simulink model "integral_backstepping"  (R2025a)
settings: Solver=VariableStepAuto  StartTime=0.0  StopTime=t_total(end)  RelTol=1e-3
StopFcn:
  | autoplot;
values from neighbouring files (symbols this model uses):
  Ib = diag([params.Ix, params.Iy, params.Iz])    [setup_mission.m]
  lin_vel_0 = [0; 0; 0]    [setup_mission.m]
  mass = params.m    [setup_mission.m]
  pos_0 = p_ref(:,1) + offset_init    [setup_mission.m]
  w_bb_0 = [0; 0; 0]    [setup_mission.m]
libraries: robotcorelib x2, uavutilslib x1
settings Model: Creator=marco  LastModifiedBy=marco

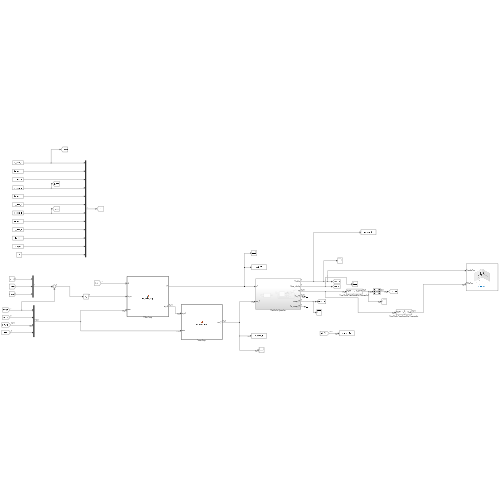
[thumbnail: Simulink's stored preview of the top-level diagram]
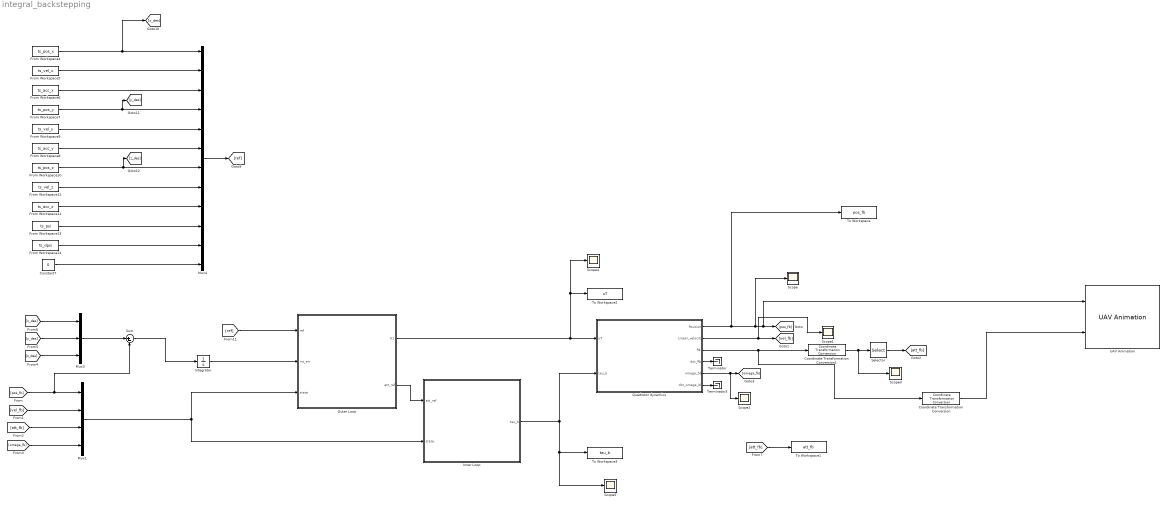
== system integral_backstepping ==
  Constant7 : Constant  Value=0
  Coordinate Transformation Conversion : robotcorelib/Coordinate Transformation Conversion  InputRepresentation=Rotation Matrix  InputEulerSequence=ZYX  ShowTrVecInputPort=on  OutputRepresentation=Quaternion  OutputEulerSequence=ZYX  ShowTrVecOutputPort=on  SimulateUsing=Interpreted execution
  Coordinate Transformation Conversion1 : robotcorelib/Coordinate Transformation Conversion  InputRepresentation=Rotation Matrix  InputEulerSequence=ZYX  ShowTrVecInputPort=on  OutputRepresentation=Euler Angles  OutputEulerSequence=ZYX  ShowTrVecOutputPort=on  SimulateUsing=Interpreted execution
  From Workspace10 : FromWorkspace  VariableName=ts_pos_z
  From Workspace11 : FromWorkspace  VariableName=ts_vel_z
  From Workspace12 : FromWorkspace  VariableName=ts_acc_z
  From Workspace13 : FromWorkspace  VariableName=ts_psi
  From Workspace14 : FromWorkspace  VariableName=ts_dpsi
  From Workspace4 : FromWorkspace  VariableName=ts_pos_x
  From Workspace5 : FromWorkspace  VariableName=ts_vel_x
  From Workspace6 : FromWorkspace  VariableName=ts_acc_x
  From Workspace7 : FromWorkspace  VariableName=ts_pos_y
  From Workspace8 : FromWorkspace  VariableName=ts_acc_y
  From Workspace9 : FromWorkspace  VariableName=ts_vel_y
  Inner Loop : MATLAB Function  TreatAsAtomicUnit=on
  Integrator : Integrator  LimitOutput=on  UpperSaturationLimit=2  LowerSaturationLimit=-2
  Mux1 : Mux
  Mux3 : Mux  Inputs=3
  Mux4 : Mux  Inputs=12
  Outer Loop : MATLAB Function  TreatAsAtomicUnit=on
  Quadrotor dynamics : Subsystem
  Scope{,1..5} (6 alike) : Scope
      Scope settings: ActiveDisplayYMinimum=-2.8808245594463218  ActiveDisplayYMaximum=14.560893195551783
      Scope1 settings: ActiveDisplayYMinimum=-1  ActiveDisplayYMaximum=1
      Scope2 settings: ActiveDisplayYMinimum=-1  ActiveDisplayYMaximum=1  DataLoggingVariableName=ScopeData2
      Scope3 settings: ActiveDisplayYMinimum=-1  ActiveDisplayYMaximum=1  DataLoggingVariableName=ScopeData3
      Scope4 settings: ActiveDisplayYMinimum=1.6033918369642832  ActiveDisplayYMaximum=12.723045351448414  DataLoggingVariableName=ScopeData4
      Scope5 settings: ActiveDisplayYMinimum=-0.020164289135421433  ActiveDisplayYMaximum=0.020163735646024  DataLoggingVariableName=ScopeData5
  Selector : Selector  InputPortWidth=3  IndexOptions=Index vector (dialog)  Indices=[3, 2, 1]  OutputSizes=1
  Sum : Sum  Inputs=|+-
  Terminator : Terminator
  Terminator3 : Terminator
  To Workspace : ToWorkspace  VariableName=pos_fb  SaveFormat=Timeseries  SampleTime=-1
  To Workspace1 : ToWorkspace  VariableName=att_fb  SaveFormat=Timeseries  SampleTime=-1
  To Workspace2 : ToWorkspace  VariableName=uT  SaveFormat=Timeseries  SampleTime=-1
  To Workspace3 : ToWorkspace  VariableName=tau_b  SaveFormat=Timeseries  SampleTime=-1
  UAV Animation : uavutilslib/UAV Animation  NumUAV=1  DynamicUAVConfig=off  UAVType=Multirotor  UAVSize=1  UAVColor=[1 0 0]  UAVTrajectoryAlpha=1  InertialZDirection=Down  RotationFormat=Quaternion  DrawMarkers=off  SampleTime=0.01
  wires:
  Quadrotor dynamics/5(omega_bb) -> [omega_fb], Scope2/1
  [pos_fb] -> Sum/2, Mux1/1
  Quadrotor dynamics/2(Linear_velocity) -> Scope1/1, [vel_fb]
  Quadrotor dynamics/4(dot_Rb) -> Terminator/1
  [omega_fb] -> Mux1/4
  Coordinate Transformation Conversion/1 -> UAV Animation/2
  [att_fb] -> Mux1/3
  Quadrotor dynamics/6(dot_omega_bb) -> Terminator3/1
  Quadrotor dynamics/3(Rb) -> Coordinate Transformation Conversion/1, Coordinate Transformation Conversion1/1
  Quadrotor dynamics/1(Position) -> To Workspace/1, Scope/1, UAV Animation/1, [pos_fb]
  Selector/1 -> [att_fb]
  Coordinate Transformation Conversion1/1 -> Selector/1, Scope3/1
  [vel_fb] -> Mux1/2
  [y_des] -> Mux3/2
  [x_des] -> Mux3/1
  [z_des] -> Mux3/3
  Mux3/1 -> Sum/1
  Mux1/1 -> Inner Loop/2(state), Outer Loop/3(state)
  Integrator/1 -> Outer Loop/2(int_err)
  Sum/1 -> Integrator/1
  [att_fb] -> To Workspace1/1
  From Workspace6/1 -> Mux4/3
  Constant7/1 -> Mux4/12
  From Workspace8/1 -> Mux4/6
  From Workspace12/1 -> Mux4/9
  From Workspace10/1 -> [z_des], Mux4/7
  Mux4/1 -> [ref]
  From Workspace4/1 -> [x_des], Mux4/1
  From Workspace14/1 -> Mux4/11
  From Workspace13/1 -> Mux4/10
  From Workspace9/1 -> Mux4/5
  From Workspace5/1 -> Mux4/2
  From Workspace7/1 -> [y_des], Mux4/4
  From Workspace11/1 -> Mux4/8
  [ref] -> Outer Loop/1(ref)
  Outer Loop/1(U1) -> Quadrotor dynamics/1(uT), Scope4/1, To Workspace2/1
  Outer Loop/2(att_ref) -> Inner Loop/1(att_ref)
  Inner Loop/1(tau_b) -> Quadrotor dynamics/2(tau_b), Scope5/1, To Workspace3/1

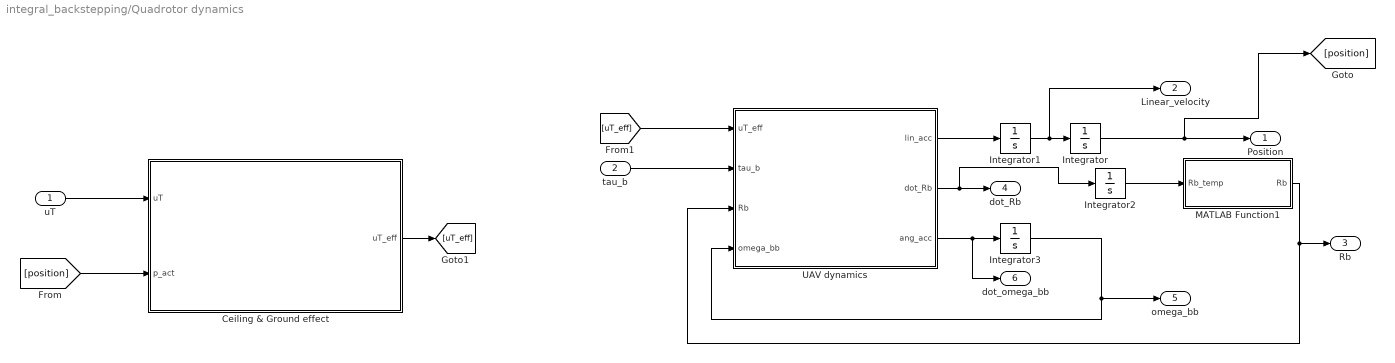
== system integral_backstepping/Quadrotor dynamics ==
  uT : Inport
  tau_b : Inport  Port=2
  Ceiling & Ground effect : MATLAB Function  TreatAsAtomicUnit=on
  Integrator : Integrator  InitialCondition=pos_0
  Integrator1 : Integrator  InitialCondition=lin_vel_0
  Integrator2 : Integrator  InitialCondition=[1 0 0; 0 1 0;0 0 1]
  Integrator3 : Integrator  InitialCondition=w_bb_0
  MATLAB Function1 : MATLAB Function  TreatAsAtomicUnit=on
  UAV dynamics : MATLAB Function  TreatAsAtomicUnit=on
  Position : Outport
  Linear_velocity : Outport  Port=2
  Rb : Outport  Port=3
  dot_Rb : Outport  Port=4
  omega_bb : Outport  Port=5
  dot_omega_bb : Outport  Port=6
  wires:
  uT/1 -> Ceiling & Ground effect/1(uT)
  Ceiling & Ground effect/1(uT_eff) -> [uT_eff]
  MATLAB Function1/1(Rb) -> Rb/1, UAV dynamics/3(Rb)
  UAV dynamics/1(lin_acc) -> Integrator1/1
  [position] -> Ceiling & Ground effect/2(p_act)
  UAV dynamics/2(dot_Rb) -> Integrator2/1, dot_Rb/1
  Integrator2/1 -> MATLAB Function1/1(Rb_temp)
  Integrator/1 -> [position], Position/1
  UAV dynamics/3(ang_acc) -> dot_omega_bb/1, Integrator3/1
  [uT_eff] -> UAV dynamics/1(uT_eff)
  Integrator3/1 -> UAV dynamics/4(omega_bb), omega_bb/1
  Integrator1/1 -> Linear_velocity/1, Integrator/1
  tau_b/1 -> UAV dynamics/2(tau_b)

== matlab function integral_backstepping/Quadrotor dynamics/Ceiling & Ground effect ==
  data: uT input; uT_eff output; p_act input
function uT_eff = aero_disturbances(uT, p_act)
% AERO_DISTURBANCES: Calcola l'effetto suolo e soffitto sulla spinta
% Riceve il comando del controller (uT) e restituisce la spinta effettiva (uT_eff)

% --- 1. PARAMETRI AMBIENTALI E DEL DRONE ---
R = 0.15;           % Raggio elica [m] (Tipico OS4)
H_room = 3.0;       % Altezza stanza [m] (Soffitto a -3.0m NED)

% Coefficienti Ceiling Effect
k1 = 6.924;
k2 = 0.03782;

% --- 2. CALCOLO DISTANZE (Frame NED) ---
z_drone = p_act(3);         % Quota attuale (negativa in volo)
d_ground = -z_drone;        % Distanza dal pavimento (z=0)
d_ceil   = H_room - d_ground; % Distanza dal soffitto (z=-3)

% Saturazione di sicurezza per evitare divisioni per zero
d_ground = max(0.05, d_ground);
d_ceil   = max(0.05, d_ceil);

% --- 3. GROUND EFFECT ---
K_ground = 1.0;
if d_ground < (2 * R)
    ratio_g = (R / (4 * d_ground))^2;
    ratio_g = min(ratio_g, 0.9); % Saturazione per evitare singolarità
    K_ground = 1 / (1 - ratio_g);
end

% --- 4. CEILING EFFECT ---
K_ceil = 1.0;
if d_ceil < (2 * R)
    term_num = (R / (d_ceil + k2))^2;
    term_den = k1;
    ratio_c  = term_num / term_den;
    ratio_c  = min(ratio_c, 0.9); % Saturazione
    K_ceil   = 1 / (1 - ratio_c);
end

% --- 5. CALCOLO SPINTA EFFETTIVA ---
K_tot = K_ground * K_ceil;
uT_eff = uT * K_tot;

end

== matlab function integral_backstepping/Outer Loop ==
  data: ref input; int_err input; U1 output; state input; params parameter; att_ref output
function [U1, att_ref] = ibs_outer_loop(ref, int_err, state, params)
% --- INTEGRAL BACKSTEPPING OUTER LOOP (POSIZIONE) ---

% --- 1. ESTRAZIONE DATI ---
x = state(1); y = state(2); z = state(3);
vx = state(4); vy = state(5); vz = state(6);
phi = state(7); theta = state(8); psi = state(9);

m = params.m;
g = params.g;

x_d = ref(1);  vx_d = ref(2);  ax_d = ref(3);
y_d = ref(4);  vy_d = ref(5);  ay_d = ref(6);
z_d = ref(7);  vz_d = ref(8);  az_d = ref(9);
psi_d = ref(10); dpsi_d = ref(11); 

int_ex = int_err(1);
int_ey = int_err(2);
int_ez = int_err(3);

% --- 2. TUNING GUADAGNI (Outer Loop) ---
% Z-Axis
Kp_z = 25.0;    
Kd_z = 25.0;    
Ki_z = 10.0;    

% XY-Plane
Kp_xy = 10.0;   
Kd_xy = 12.0;   
Ki_xy = 2.0;    

% --- 3. CONTROLLO POSIZIONE (PID Virtuale) ---
ex = x_d - x;  dex = vx_d - vx;
ey = y_d - y;  dey = vy_d - vy;
ez = z_d - z;  dez = vz_d - vz;

mu_x = ax_d + Kd_xy * dex + Kp_xy * ex + Ki_xy * int_ex;
mu_y = ay_d + Kd_xy * dey + Kp_xy * ey + Ki_xy * int_ey;
mu_z = az_d + Kd_z  * dez + Kp_z  * ez + Ki_z  * int_ez;

% --- 4. CALCOLO SPINTA TOTALE (U1) ---
term_z = g - mu_z;
den_z = cos(phi) * cos(theta);

% Protezione divisione per zero (coseno)
if abs(den_z) < 0.1
    den_z = sign(den_z) * 0.1; 
    if den_z == 0, den_z = 0.1; end
end

U1 = (m * term_z) / den_z;
U1 = max(0, U1); % Saturazione Fisica       

% --- PROTEZIONE SINGOLARITÀ (Ceiling Effect) ---
min_thrust_calc = 2.5; 
if U1 < min_thrust_calc
    U1_safe = min_thrust_calc; 
else
    U1_safe = U1;
end

% --- 5. INVERSIONE ANGOLI ---
comm_x = (m / U1_safe) * mu_x;
comm_y = (m / U1_safe) * mu_y;

theta_d_raw = -(comm_x * cos(psi) + comm_y * sin(psi));
phi_d_raw   = comm_y * cos(psi) - comm_x * sin(psi);

% Saturazione Angoli (Anti-Ribaltamento)
max_angle = 0.6; 
theta_d = max(min(theta_d_raw, max_angle), -max_angle);
phi_d   = max(min(phi_d_raw, max_angle), -max_angle);

% --- 6. OUTPUT VERSO L'INNER LOOP ---
att_ref = [phi_d; theta_d; psi_d; dpsi_d];

end

== matlab function integral_backstepping/Inner Loop ==
  data: att_ref input; tau_b output; state input; params parameter
function tau_b  = ibs_inner_loop(att_ref, state, params)
% --- INTEGRAL BACKSTEPPING INNER LOOP (ATTITUDINE) ---

% --- 1. ESTRAZIONE DATI ---
phi_d = att_ref(1);
theta_d = att_ref(2);
psi_d = att_ref(3);
dpsi_d = att_ref(4);

phi = state(7); theta = state(8); psi = state(9);
p = state(10); q = state(11); r = state(12);

Ix = params.Ix; Iy = params.Iy; Iz = params.Iz;

% --- 2. TUNING GUADAGNI (Inner Loop) ---
Kp_att = 70.0;  
Kd_att = 22.0;  

% --- 3. CONTROLLO ATTITUDINE (PD) ---
e_phi = phi_d - phi;     
de_phi = 0 - p;  

e_theta = theta_d - theta; 
de_theta = 0 - q;

e_psi = psi_d - psi;     
de_psi = dpsi_d - r;


% Legge di controllo per i momenti
U2 = Ix * (Kp_att * e_phi + Kd_att * de_phi);
U3 = Iy * (Kp_att * e_theta  + Kd_att * de_theta);
U4 = Iz * (Kp_att * e_psi + Kd_att * de_psi);

% --- 4. OUTPUT ---
tau_b = [U2; U3; U4];

end

== matlab function integral_backstepping/Quadrotor dynamics/UAV dynamics ==
  data: uT_eff input size=1; tau_b input size=3; lin_acc output size=3; Rb input size=[3,3]; omega_bb input size=3; dot_Rb output size=[3,3]; ang_acc output size=3; mass parameter size=1; Ib parameter size=[3,3]
function [lin_acc, dot_Rb, ang_acc] = uav_dynamics(uT_eff, tau_b, Rb, omega_bb, mass, Ib)
% UAV_DYNAMICS: Modello cinematico e dinamico del quadricottero.
% Ingressi:
% - uT_eff: Spinta totale effettiva (già perturbata dall'aerodinamica)
% - tau_b, Rb, omega_bb, mass (nominale), Ib

% --- 1. INCERTEZZA PARAMETRICA ---
% Massa reale per la simulazione (Robustness check: +40% rispetto al modello nominale)
m_real = mass * 1.4; 

g = 9.81;
e3 = [0; 0; 1];

% --- 2. DINAMICA TRASLAZIONALE ---
% Forza Spinta nel frame Inerziale (Ruotata da Rb)
% Nota: Dividiamo per m_real perché questa è la dinamica "vera" del sistema
Thrust_Inertial = (uT_eff / m_real) * Rb * e3;

% Accelerazione Lineare (NED: g positiva verso il basso)
lin_acc = g * e3 - Thrust_Inertial; 

% --- 3. DINAMICA ROTAZIONALE ---
dot_Rb = Rb * skew(omega_bb);

% Momenti: Si assume che i disturbi aerodinamici sui momenti siano trascurabili
ang_acc = Ib \ (-skew(omega_bb) * Ib * omega_bb + tau_b);

end

% --- Funzione di supporto ---
function S = skew(v)
if(numel(v)~= 1)
    S= [0 -v(3) v(2); v(3) 0 -v(1); -v(2) v(1) 0];
else
    S= zeros(3);
end
end

== matlab function integral_backstepping/Quadrotor dynamics/MATLAB Function1 ==
  data: Rb_temp input; Rb output
function Rb = fcn(Rb_temp)
    [U,S,V] = svd(Rb_temp);
    sigma = det(U*V');
    S_ = diag([1 1 sigma]);

    Rb = U*S_*V';
end
